simulink model "MK_elem_cl"  (R2025b)
settings: Solver=VariableStepAuto  StartTime=0.0  StopTime=10.0  RelTol=1e-3
undefined symbols (not defined in the file): invio, Z
libraries: cstblocks x2
settings Model: Creator=d.alazard  LastModifiedBy=andre
settings SolverCC: AlgebraicLoopSolver=TrustRegion
settings DebuggingCC: AlgebraicLoopMsg=none  UnconnectedInputMsg=warning  UnconnectedOutputMsg=warning  UnconnectedLineMsg=warning
settings ModelReferenceCC: EnableRefExpFcnMdlSchedulingChecks=on
settings RTWCC: GPUComputeCapability=3.5  DLArmComputeVersion=19.05

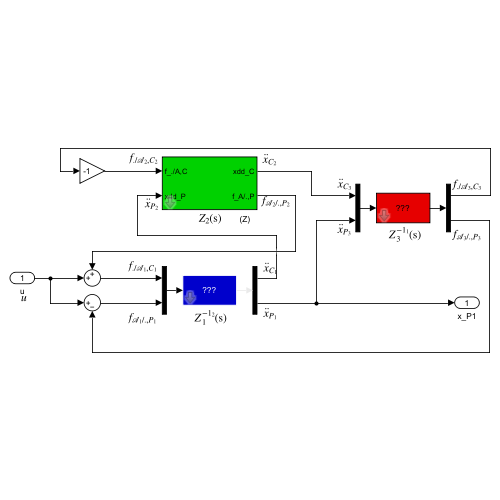
[thumbnail: Simulink's stored preview of the top-level diagram]
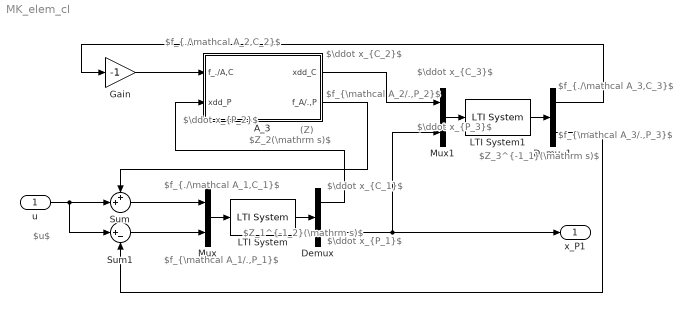
== system MK_elem_cl ==
  note: (Z)
  note: $u$
  note: $f_{\mathcal A_1/.,P_1}$
  note: $\ddot x_{P_1}$
  note: $\ddot x_{C_1}$
  note: $\ddot x_{P_2}$
  note: $\ddot x_{P_3}$
  note: $\ddot x_{C_2}$
  note: $\ddot x_{C_3}$
  note: $f_{\mathcal A_2/.,P_2}$
  note: $f_{\mathcal A_3/.,P_3}$
  note: $f_{./\mathcal A_1,C_1}$
  note: $f_{./\mathcal A_2,C_2}$
  note: $f_{./\mathcal A_3,C_3}$
  note: $Z_2(\mathrm s)$
  note: $Z_1^{-1_2}(\mathrm s)$
  note: $Z_3^{-1_1}(\mathrm s)$
  u : Inport
  A_3 : Subsystem  mask(Spring mass system){k=1, m_P=2, m_C=3}
      mask prompts: k "stiffness k (N/m)"; m_P "mass m_P (Kg)"; m_C "mass m_C (Kg)"
      mask help: TITOP model of the spring-mass system
  Demux : Demux  Outputs=2
  Demux1 : Demux  Outputs=2
  Gain : Gain  Gain=-1
  LTI System : cstblocks/LTI System  sys=invio(Z,2)  IC=[]  PadeOrder=0
  LTI System1 : cstblocks/LTI System  sys=invio(Z,1)  IC=[]  PadeOrder=0
  Mux : Mux  Inputs=2
  Mux1 : Mux  Inputs=2
  Sum : Sum  Inputs=++|
  Sum1 : Sum  Inputs=|+-
  x_P1 : Outport
  wires:
  Mux/1 -> LTI System/1
  LTI System/1 -> Demux/1
  Sum/1 -> Mux/1
  Demux/2 -> Mux1/2, x_P1/1
  LTI System1/1 -> Demux1/1
  Mux1/1 -> LTI System1/1
  Demux/1 -> A_3/2(xdd_P)
  A_3/2(f_A/.,P) -> Sum/1
  u/1 -> Sum1/1, Sum/2
  Sum1/1 -> Mux/2
  A_3/1(xdd_C) -> Mux1/1
  Demux1/2 -> Sum1/2
  Demux1/1 -> Gain/1
  Gain/1 -> A_3/1(f_./A,C)

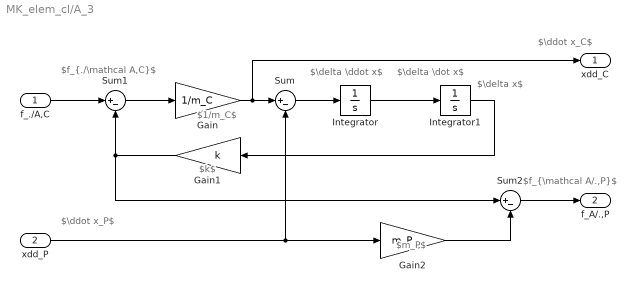
== system MK_elem_cl/A_3 ==
  note: $\delta x$
  note: $\delta \dot x$
  note: $\delta \ddot x$
  note: $\ddot x_P$
  note: $\ddot x_C$
  note: $f_{\mathcal A/.,P}$
  note: $f_{./\mathcal A,C}$
  note: $1/m_C$
  note: $k$
  note: $m_P$
  f_./A,C : Inport
  xdd_P : Inport  Port=2
  Gain : Gain  Gain=1/m_C
  Gain1 : Gain  Gain=k
  Gain2 : Gain  Gain=m_P
  Integrator : Integrator
  Integrator1 : Integrator
  Sum : Sum  Inputs=|+-
  Sum1 : Sum  Inputs=|+-
  Sum2 : Sum  Inputs=|+-
  xdd_C : Outport
  f_A/.,P : Outport  Port=2
  wires:
  Sum2/1 -> f_A/.,P/1
  Integrator/1 -> Integrator1/1
  Gain1/1 -> Sum2/1, Sum1/2
  Sum1/1 -> Gain/1
  Sum/1 -> Integrator/1
  xdd_P/1 -> Gain2/1, Sum/2
  Integrator1/1 -> Gain1/1
  Gain/1 -> xdd_C/1, Sum/1
  Gain2/1 -> Sum2/2
  f_./A,C/1 -> Sum1/1
